simulink model "ADIA"  (R2018b)
settings: Solver=FixedStepDiscrete  StartTime=0.0  StopTime=10.0  FixedStep=0.02  RelTol=1e-3
undefined symbols (not defined in the file or in its folder): ACC_State_Active, ACC_State_BrakeOnly, ACC_State_Suspended, ACC_State_WaitingRise, ADAS_AEBBrakingProg, ADAS_DeclControlReq, ADAS_DriveOff, ADAS_ESCHoldReq_NotHold, ADASDecType_ACC, ADASDecType_AEB, ADIA_ACC_Acceleration_OOR_DecCount_C, ADIA_ACC_Acceleration_OOR_Duration_C, ADIA_ACC_Acceleration_OOR_IncCount_C, ADIA_ACC_Acceleration_OOR_LLim_C, ADIA_ACC_Acceleration_OOR_ULim_C, ADIA_ACC_AccelTrqReq_MixedDia_ULim_C, ADIA_ACC_AccelTrqReq_ULim_C, ADIA_ACC_Deceleration_Mixed_ULim_C, ADIA_ACC_Deceleration_OOR_DecCount_C, ADIA_ACC_Deceleration_OOR_Duration_C, ADIA_ACC_Deceleration_OOR_IncCount_C, ADIA_ACC_Deceleration_OOR_LLim_C, ADIA_ACC_Deceleration_OOR_ULim_C, ADIA_ACC_DriveOff_Distance_C, ADIA_ACC_DriveOff_TimeLim_C, ADIA_ACC_ReqMixed_DecCount_C, ADIA_ACC_ReqMixed_Duration_C, ADIA_ACC_ReqMixed_IncCount_C, ADIA_AccPedalRaw_MaxLim_C, ADIA_AccPedalRaw_MinLim_C, ADIA_ADAS_HoldDecReq_Set_C, ADIA_ADAS_HoldRConfirm_TimeLim_C, ADIA_ADAS_HoldVehSpd_Lim_C, ADIA_AEB_VehSpdDec_LLim_C, ADIA_AEB_VehSpdDec_ULim_C, ADIA_ASWFault_OvrdEn_C, ADIA_ASWFault_OvrdValue_C, ADIA_BatteryOutOfRange_DecCount_C, ADIA_BatteryOutOfRange_Duration_C, ADIA_BatteryOutOfRange_IncCount_C, ADIA_BattVolt_MaxLim_C, ADIA_BattVolt_MinLim_C, ADIA_BCM3_33C_InvBrkLight_DecCount_C, ADIA_BCM3_33C_InvBrkLight_Duration_C, ADIA_BCM3_33C_InvBrkLight_IncCount_C, ADIA_BCM_BattVolt_OvrdEn_C, ADIA_BCM_BattVolt_OvrdVal_C, ADIA_BCM_BrakeLampStaus_OvrdEn_C, ADIA_BCM_BrakeLampStaus_OvrdVal_C, ADIA_BCM_CHMSLStaus_OvrdEn_C, ADIA_BCM_CHMSLStaus_OvrdVal_C, ADIA_BCM_LeftTurnSwSt_OvrdEn_C, ADIA_BCM_LeftTurnSwSt_OvrdVal_C, ADIA_BCM_RightTurnSwSt_OvrdEn_C, ADIA_BCM_RightTurnSwSt_OvrdVal_C, ADIA_BCM_TurnSwFailure_DecCount_C, ADIA_BCM_TurnSwFailure_Duration_C, ADIA_BCM_TurnSwFailure_IncCount_C, ADIA_BSWFault_Ignore_C, ADIA_BSWFault_OvrdEn_C ... (+281)
libraries: simulink x208
(part 7 of 10)

== system ADIA/ADAS_Diagnostics/Diagnostics_Processing/Rationality_Diagnostics/ESC3_121_InvOorVehStand/Counter&Latch ==
  incrcondition : Inport
  incrvalue : Inport  Port=2
  decrcondition : Inport  Port=3
  decvalue : Inport  Port=4
  maxlimit : Inport  Port=5
  reset : Inport  Port=6
  LatchResetCounterVal : Inport  Port=7
  "Latch " : Subsystem
  Relational Operator16 : RelationalOperator  Operator=<=  OutDataTypeStr=boolean  RndMeth=Simplest
  Timer1 : Subsystem
  Out1 : Outport
  wires:
  Timer1/2(counter_status) -> "Latch "/1(Input)
  Timer1/1(counter out) -> Relational Operator16/1
  LatchResetCounterVal/1 -> Relational Operator16/2
  incrcondition/1 -> Timer1/1(incrcondition)
  incrvalue/1 -> Timer1/2(incrvalue)
  Relational Operator16/1 -> "Latch "/2(Latch Reset)
  "Latch "/1(Output) -> Out1/1
  maxlimit/1 -> Timer1/5(maxlimit)
  decrcondition/1 -> Timer1/3(decrcondition)
  reset/1 -> Timer1/6(reset)
  decvalue/1 -> Timer1/4(decvalue)

== system ADIA/ADAS_Diagnostics/Diagnostics_Processing/Rationality_Diagnostics/ESC5_122_InvOorLatAccel/Counter&Latch ==
  incrcondition : Inport
  incrvalue : Inport  Port=2
  decrcondition : Inport  Port=3
  decvalue : Inport  Port=4
  maxlimit : Inport  Port=5
  reset : Inport  Port=6
  LatchResetCounterVal : Inport  Port=7
  "Latch " : Subsystem
  Relational Operator16 : RelationalOperator  Operator=<=  OutDataTypeStr=boolean  RndMeth=Simplest
  Timer1 : Subsystem
  Out1 : Outport
  wires:
  Timer1/2(counter_status) -> "Latch "/1(Input)
  Timer1/1(counter out) -> Relational Operator16/1
  LatchResetCounterVal/1 -> Relational Operator16/2
  incrcondition/1 -> Timer1/1(incrcondition)
  incrvalue/1 -> Timer1/2(incrvalue)
  Relational Operator16/1 -> "Latch "/2(Latch Reset)
  "Latch "/1(Output) -> Out1/1
  maxlimit/1 -> Timer1/5(maxlimit)
  decrcondition/1 -> Timer1/3(decrcondition)
  reset/1 -> Timer1/6(reset)
  decvalue/1 -> Timer1/4(decvalue)

== system ADIA/ADAS_Diagnostics/Diagnostics_Processing/Rationality_Diagnostics/ESC5_122_InvOorLongiAccel/Counter&Latch ==
  incrcondition : Inport
  incrvalue : Inport  Port=2
  decrcondition : Inport  Port=3
  decvalue : Inport  Port=4
  maxlimit : Inport  Port=5
  reset : Inport  Port=6
  LatchResetCounterVal : Inport  Port=7
  "Latch " : Subsystem
  Relational Operator16 : RelationalOperator  Operator=<=  OutDataTypeStr=boolean  RndMeth=Simplest
  Timer1 : Subsystem
  Out1 : Outport
  wires:
  Timer1/2(counter_status) -> "Latch "/1(Input)
  Timer1/1(counter out) -> Relational Operator16/1
  LatchResetCounterVal/1 -> Relational Operator16/2
  incrcondition/1 -> Timer1/1(incrcondition)
  incrvalue/1 -> Timer1/2(incrvalue)
  Relational Operator16/1 -> "Latch "/2(Latch Reset)
  "Latch "/1(Output) -> Out1/1
  maxlimit/1 -> Timer1/5(maxlimit)
  decrcondition/1 -> Timer1/3(decrcondition)
  reset/1 -> Timer1/6(reset)
  decvalue/1 -> Timer1/4(decvalue)

== system ADIA/ADAS_Diagnostics/Diagnostics_Processing/Rationality_Diagnostics/ESC5_122_InvOorStaticSlope/Counter&Latch ==
  incrcondition : Inport
  incrvalue : Inport  Port=2
  decrcondition : Inport  Port=3
  decvalue : Inport  Port=4
  maxlimit : Inport  Port=5
  reset : Inport  Port=6
  LatchResetCounterVal : Inport  Port=7
  "Latch " : Subsystem
  Relational Operator16 : RelationalOperator  Operator=<=  OutDataTypeStr=boolean  RndMeth=Simplest
  Timer1 : Subsystem
  Out1 : Outport
  wires:
  Timer1/2(counter_status) -> "Latch "/1(Input)
  Timer1/1(counter out) -> Relational Operator16/1
  LatchResetCounterVal/1 -> Relational Operator16/2
  incrcondition/1 -> Timer1/1(incrcondition)
  incrvalue/1 -> Timer1/2(incrvalue)
  Relational Operator16/1 -> "Latch "/2(Latch Reset)
  "Latch "/1(Output) -> Out1/1
  maxlimit/1 -> Timer1/5(maxlimit)
  decrcondition/1 -> Timer1/3(decrcondition)
  reset/1 -> Timer1/6(reset)
  decvalue/1 -> Timer1/4(decvalue)

== system ADIA/ADAS_Diagnostics/Diagnostics_Processing/Rationality_Diagnostics/ESC5_122_InvOorYawRate/Counter&Latch ==
  incrcondition : Inport
  incrvalue : Inport  Port=2
  decrcondition : Inport  Port=3
  decvalue : Inport  Port=4
  maxlimit : Inport  Port=5
  reset : Inport  Port=6
  LatchResetCounterVal : Inport  Port=7
  "Latch " : Subsystem
  Relational Operator16 : RelationalOperator  Operator=<=  OutDataTypeStr=boolean  RndMeth=Simplest
  Timer1 : Subsystem
  Out1 : Outport
  wires:
  Timer1/2(counter_status) -> "Latch "/1(Input)
  Timer1/1(counter out) -> Relational Operator16/1
  LatchResetCounterVal/1 -> Relational Operator16/2
  incrcondition/1 -> Timer1/1(incrcondition)
  incrvalue/1 -> Timer1/2(incrvalue)
  Relational Operator16/1 -> "Latch "/2(Latch Reset)
  "Latch "/1(Output) -> Out1/1
  maxlimit/1 -> Timer1/5(maxlimit)
  decrcondition/1 -> Timer1/3(decrcondition)
  reset/1 -> Timer1/6(reset)
  decvalue/1 -> Timer1/4(decvalue)

== system ADIA/ADAS_Diagnostics/Diagnostics_Processing/Rationality_Diagnostics/ESC6_123_InvOorDynSlope/Counter&Latch ==
  incrcondition : Inport
  incrvalue : Inport  Port=2
  decrcondition : Inport  Port=3
  decvalue : Inport  Port=4
  maxlimit : Inport  Port=5
  reset : Inport  Port=6
  LatchResetCounterVal : Inport  Port=7
  "Latch " : Subsystem
  Relational Operator16 : RelationalOperator  Operator=<=  OutDataTypeStr=boolean  RndMeth=Simplest
  Timer1 : Subsystem
  Out1 : Outport
  wires:
  Timer1/2(counter_status) -> "Latch "/1(Input)
  Timer1/1(counter out) -> Relational Operator16/1
  LatchResetCounterVal/1 -> Relational Operator16/2
  incrcondition/1 -> Timer1/1(incrcondition)
  incrvalue/1 -> Timer1/2(incrvalue)
  Relational Operator16/1 -> "Latch "/2(Latch Reset)
  "Latch "/1(Output) -> Out1/1
  maxlimit/1 -> Timer1/5(maxlimit)
  decrcondition/1 -> Timer1/3(decrcondition)
  reset/1 -> Timer1/6(reset)
  decvalue/1 -> Timer1/4(decvalue)

== system ADIA/ADAS_Diagnostics/Diagnostics_Processing/Rationality_Diagnostics/ESC6_123_InvUnfilYawRate/Counter&Latch ==
  incrcondition : Inport
  incrvalue : Inport  Port=2
  decrcondition : Inport  Port=3
  decvalue : Inport  Port=4
  maxlimit : Inport  Port=5
  reset : Inport  Port=6
  LatchResetCounterVal : Inport  Port=7
  "Latch " : Subsystem
  Relational Operator16 : RelationalOperator  Operator=<=  OutDataTypeStr=boolean  RndMeth=Simplest
  Timer1 : Subsystem
  Out1 : Outport
  wires:
  Timer1/2(counter_status) -> "Latch "/1(Input)
  Timer1/1(counter out) -> Relational Operator16/1
  LatchResetCounterVal/1 -> Relational Operator16/2
  incrcondition/1 -> Timer1/1(incrcondition)
  incrvalue/1 -> Timer1/2(incrvalue)
  Relational Operator16/1 -> "Latch "/2(Latch Reset)
  "Latch "/1(Output) -> Out1/1
  maxlimit/1 -> Timer1/5(maxlimit)
  decrcondition/1 -> Timer1/3(decrcondition)
  reset/1 -> Timer1/6(reset)
  decvalue/1 -> Timer1/4(decvalue)

== system ADIA/ADAS_Diagnostics/Diagnostics_Processing/Rationality_Diagnostics/ESC6_123_InvVehDriDirec/Counter&Latch ==
  incrcondition : Inport
  incrvalue : Inport  Port=2
  decrcondition : Inport  Port=3
  decvalue : Inport  Port=4
  maxlimit : Inport  Port=5
  reset : Inport  Port=6
  LatchResetCounterVal : Inport  Port=7
  "Latch " : Subsystem
  Relational Operator16 : RelationalOperator  Operator=<=  OutDataTypeStr=boolean  RndMeth=Simplest
  Timer1 : Subsystem
  Out1 : Outport
  wires:
  Timer1/2(counter_status) -> "Latch "/1(Input)
  Timer1/1(counter out) -> Relational Operator16/1
  LatchResetCounterVal/1 -> Relational Operator16/2
  incrcondition/1 -> Timer1/1(incrcondition)
  incrvalue/1 -> Timer1/2(incrvalue)
  Relational Operator16/1 -> "Latch "/2(Latch Reset)
  "Latch "/1(Output) -> Out1/1
  maxlimit/1 -> Timer1/5(maxlimit)
  decrcondition/1 -> Timer1/3(decrcondition)
  reset/1 -> Timer1/6(reset)
  decvalue/1 -> Timer1/4(decvalue)

== system ADIA/ADAS_Diagnostics/Diagnostics_Processing/Rationality_Diagnostics/ESC6_123_InvVehHoldStas/Counter&Latch ==
  incrcondition : Inport
  incrvalue : Inport  Port=2
  decrcondition : Inport  Port=3
  decvalue : Inport  Port=4
  maxlimit : Inport  Port=5
  reset : Inport  Port=6
  LatchResetCounterVal : Inport  Port=7
  "Latch " : Subsystem
  Relational Operator16 : RelationalOperator  Operator=<=  OutDataTypeStr=boolean  RndMeth=Simplest
  Timer1 : Subsystem
  Out1 : Outport
  wires:
  Timer1/2(counter_status) -> "Latch "/1(Input)
  Timer1/1(counter out) -> Relational Operator16/1
  LatchResetCounterVal/1 -> Relational Operator16/2
  incrcondition/1 -> Timer1/1(incrcondition)
  incrvalue/1 -> Timer1/2(incrvalue)
  Relational Operator16/1 -> "Latch "/2(Latch Reset)
  "Latch "/1(Output) -> Out1/1
  maxlimit/1 -> Timer1/5(maxlimit)
  decrcondition/1 -> Timer1/3(decrcondition)
  reset/1 -> Timer1/6(reset)
  decvalue/1 -> Timer1/4(decvalue)

== system ADIA/ADAS_Diagnostics/Diagnostics_Processing/Rationality_Diagnostics/FRadar_FaultState/Counter&Latch ==
  incrcondition : Inport
  incrvalue : Inport  Port=2
  decrcondition : Inport  Port=3
  decvalue : Inport  Port=4
  maxlimit : Inport  Port=5
  reset : Inport  Port=6
  LatchResetCounterVal : Inport  Port=7
  "Latch " : Subsystem
  Relational Operator16 : RelationalOperator  Operator=<=  OutDataTypeStr=boolean  RndMeth=Simplest
  Timer1 : Subsystem
  Out1 : Outport
  wires:
  Timer1/2(counter_status) -> "Latch "/1(Input)
  Timer1/1(counter out) -> Relational Operator16/1
  LatchResetCounterVal/1 -> Relational Operator16/2
  incrcondition/1 -> Timer1/1(incrcondition)
  incrvalue/1 -> Timer1/2(incrvalue)
  Relational Operator16/1 -> "Latch "/2(Latch Reset)
  "Latch "/1(Output) -> Out1/1
  maxlimit/1 -> Timer1/5(maxlimit)
  decrcondition/1 -> Timer1/3(decrcondition)
  reset/1 -> Timer1/6(reset)
  decvalue/1 -> Timer1/4(decvalue)

== system ADIA/ADAS_Diagnostics/Diagnostics_Processing/Rationality_Diagnostics/MP5_366_OorAEBButton/Counter&Latch ==
  incrcondition : Inport
  incrvalue : Inport  Port=2
  decrcondition : Inport  Port=3
  decvalue : Inport  Port=4
  maxlimit : Inport  Port=5
  reset : Inport  Port=6
  LatchResetCounterVal : Inport  Port=7
  "Latch " : Subsystem
  Relational Operator16 : RelationalOperator  Operator=<=  OutDataTypeStr=boolean  RndMeth=Simplest
  Timer1 : Subsystem
  Out1 : Outport
  wires:
  Timer1/2(counter_status) -> "Latch "/1(Input)
  Timer1/1(counter out) -> Relational Operator16/1
  LatchResetCounterVal/1 -> Relational Operator16/2
  incrcondition/1 -> Timer1/1(incrcondition)
  incrvalue/1 -> Timer1/2(incrvalue)
  Relational Operator16/1 -> "Latch "/2(Latch Reset)
  "Latch "/1(Output) -> Out1/1
  maxlimit/1 -> Timer1/5(maxlimit)
  decrcondition/1 -> Timer1/3(decrcondition)
  reset/1 -> Timer1/6(reset)
  decvalue/1 -> Timer1/4(decvalue)

== system ADIA/ADAS_Diagnostics/Diagnostics_Processing/Rationality_Diagnostics/MP5_366_OorFCWButton/Counter&Latch ==
  incrcondition : Inport
  incrvalue : Inport  Port=2
  decrcondition : Inport  Port=3
  decvalue : Inport  Port=4
  maxlimit : Inport  Port=5
  reset : Inport  Port=6
  LatchResetCounterVal : Inport  Port=7
  "Latch " : Subsystem
  Relational Operator16 : RelationalOperator  Operator=<=  OutDataTypeStr=boolean  RndMeth=Simplest
  Timer1 : Subsystem
  Out1 : Outport
  wires:
  Timer1/2(counter_status) -> "Latch "/1(Input)
  Timer1/1(counter out) -> Relational Operator16/1
  LatchResetCounterVal/1 -> Relational Operator16/2
  incrcondition/1 -> Timer1/1(incrcondition)
  incrvalue/1 -> Timer1/2(incrvalue)
  Relational Operator16/1 -> "Latch "/2(Latch Reset)
  "Latch "/1(Output) -> Out1/1
  maxlimit/1 -> Timer1/5(maxlimit)
  decrcondition/1 -> Timer1/3(decrcondition)
  reset/1 -> Timer1/6(reset)
  decvalue/1 -> Timer1/4(decvalue)

== system ADIA/ADAS_Diagnostics/Diagnostics_Processing/Rationality_Diagnostics/MP5_413_OorISAMode/Counter&Latch ==
  incrcondition : Inport
  incrvalue : Inport  Port=2
  decrcondition : Inport  Port=3
  decvalue : Inport  Port=4
  maxlimit : Inport  Port=5
  reset : Inport  Port=6
  LatchResetCounterVal : Inport  Port=7
  "Latch " : Subsystem
  Relational Operator16 : RelationalOperator  Operator=<=  OutDataTypeStr=boolean  RndMeth=Simplest
  Timer1 : Subsystem
  Out1 : Outport
  wires:
  Timer1/2(counter_status) -> "Latch "/1(Input)
  Timer1/1(counter out) -> Relational Operator16/1
  LatchResetCounterVal/1 -> Relational Operator16/2
  incrcondition/1 -> Timer1/1(incrcondition)
  incrvalue/1 -> Timer1/2(incrvalue)
  Relational Operator16/1 -> "Latch "/2(Latch Reset)
  "Latch "/1(Output) -> Out1/1
  maxlimit/1 -> Timer1/5(maxlimit)
  decrcondition/1 -> Timer1/3(decrcondition)
  reset/1 -> Timer1/6(reset)
  decvalue/1 -> Timer1/4(decvalue)

== system ADIA/ADAS_Diagnostics/Diagnostics_Processing/Rationality_Diagnostics/MP5_413_OorLKAMode/Counter&Latch ==
  incrcondition : Inport
  incrvalue : Inport  Port=2
  decrcondition : Inport  Port=3
  decvalue : Inport  Port=4
  maxlimit : Inport  Port=5
  reset : Inport  Port=6
  LatchResetCounterVal : Inport  Port=7
  "Latch " : Subsystem
  Relational Operator16 : RelationalOperator  Operator=<=  OutDataTypeStr=boolean  RndMeth=Simplest
  Timer1 : Subsystem
  Out1 : Outport
  wires:
  Timer1/2(counter_status) -> "Latch "/1(Input)
  Timer1/1(counter out) -> Relational Operator16/1
  LatchResetCounterVal/1 -> Relational Operator16/2
  incrcondition/1 -> Timer1/1(incrcondition)
  incrvalue/1 -> Timer1/2(incrvalue)
  Relational Operator16/1 -> "Latch "/2(Latch Reset)
  "Latch "/1(Output) -> Out1/1
  maxlimit/1 -> Timer1/5(maxlimit)
  decrcondition/1 -> Timer1/3(decrcondition)
  reset/1 -> Timer1/6(reset)
  decvalue/1 -> Timer1/4(decvalue)

== system ADIA/ADAS_Diagnostics/Diagnostics_Processing/Rationality_Diagnostics/SAS_A5_InvOorSteAngle/Counter&Latch ==
  incrcondition : Inport
  incrvalue : Inport  Port=2
  decrcondition : Inport  Port=3
  decvalue : Inport  Port=4
  maxlimit : Inport  Port=5
  reset : Inport  Port=6
  LatchResetCounterVal : Inport  Port=7
  "Latch " : Subsystem
  Relational Operator16 : RelationalOperator  Operator=<=  OutDataTypeStr=boolean  RndMeth=Simplest
  Timer1 : Subsystem
  Out1 : Outport
  wires:
  Timer1/2(counter_status) -> "Latch "/1(Input)
  Timer1/1(counter out) -> Relational Operator16/1
  LatchResetCounterVal/1 -> Relational Operator16/2
  incrcondition/1 -> Timer1/1(incrcondition)
  incrvalue/1 -> Timer1/2(incrvalue)
  Relational Operator16/1 -> "Latch "/2(Latch Reset)
  "Latch "/1(Output) -> Out1/1
  maxlimit/1 -> Timer1/5(maxlimit)
  decrcondition/1 -> Timer1/3(decrcondition)
  reset/1 -> Timer1/6(reset)
  decvalue/1 -> Timer1/4(decvalue)

== system ADIA/ADAS_Diagnostics/Diagnostics_Processing/Rationality_Diagnostics/SAS_A5_InvRotSpeed/Counter&Latch ==
  incrcondition : Inport
  incrvalue : Inport  Port=2
  decrcondition : Inport  Port=3
  decvalue : Inport  Port=4
  maxlimit : Inport  Port=5
  reset : Inport  Port=6
  LatchResetCounterVal : Inport  Port=7
  "Latch " : Subsystem
  Relational Operator16 : RelationalOperator  Operator=<=  OutDataTypeStr=boolean  RndMeth=Simplest
  Timer1 : Subsystem
  Out1 : Outport
  wires:
  Timer1/2(counter_status) -> "Latch "/1(Input)
  Timer1/1(counter out) -> Relational Operator16/1
  LatchResetCounterVal/1 -> Relational Operator16/2
  incrcondition/1 -> Timer1/1(incrcondition)
  incrvalue/1 -> Timer1/2(incrvalue)
  Relational Operator16/1 -> "Latch "/2(Latch Reset)
  "Latch "/1(Output) -> Out1/1
  maxlimit/1 -> Timer1/5(maxlimit)
  decrcondition/1 -> Timer1/3(decrcondition)
  reset/1 -> Timer1/6(reset)
  decvalue/1 -> Timer1/4(decvalue)

== system ADIA/ADAS_Diagnostics/Diagnostics_Processing/Rationality_Diagnostics/SCC_309_OorACCButton/Counter&Latch ==
  incrcondition : Inport
  incrvalue : Inport  Port=2
  decrcondition : Inport  Port=3
  decvalue : Inport  Port=4
  maxlimit : Inport  Port=5
  reset : Inport  Port=6
  LatchResetCounterVal : Inport  Port=7
  "Latch " : Subsystem
  Relational Operator16 : RelationalOperator  Operator=<=  OutDataTypeStr=boolean  RndMeth=Simplest
  Timer1 : Subsystem
  Out1 : Outport
  wires:
  Timer1/2(counter_status) -> "Latch "/1(Input)
  Timer1/1(counter out) -> Relational Operator16/1
  LatchResetCounterVal/1 -> Relational Operator16/2
  incrcondition/1 -> Timer1/1(incrcondition)
  incrvalue/1 -> Timer1/2(incrvalue)
  Relational Operator16/1 -> "Latch "/2(Latch Reset)
  "Latch "/1(Output) -> Out1/1
  maxlimit/1 -> Timer1/5(maxlimit)
  decrcondition/1 -> Timer1/3(decrcondition)
  reset/1 -> Timer1/6(reset)
  decvalue/1 -> Timer1/4(decvalue)

== system ADIA/ADAS_Diagnostics/Diagnostics_Processing/Rationality_Diagnostics/Subsystem1/Counter&Latch ==
  incrcondition : Inport
  incrvalue : Inport  Port=2
  decrcondition : Inport  Port=3
  decvalue : Inport  Port=4
  maxlimit : Inport  Port=5
  reset : Inport  Port=6
  LatchResetCounterVal : Inport  Port=7
  "Latch " : Subsystem
  Relational Operator16 : RelationalOperator  Operator=<=  OutDataTypeStr=boolean  RndMeth=Simplest
  Timer1 : Subsystem
  Out1 : Outport
  wires:
  Timer1/2(counter_status) -> "Latch "/1(Input)
  Timer1/1(counter out) -> Relational Operator16/1
  LatchResetCounterVal/1 -> Relational Operator16/2
  incrcondition/1 -> Timer1/1(incrcondition)
  incrvalue/1 -> Timer1/2(incrvalue)
  Relational Operator16/1 -> "Latch "/2(Latch Reset)
  "Latch "/1(Output) -> Out1/1
  maxlimit/1 -> Timer1/5(maxlimit)
  decrcondition/1 -> Timer1/3(decrcondition)
  reset/1 -> Timer1/6(reset)
  decvalue/1 -> Timer1/4(decvalue)

== system ADIA/ADAS_Diagnostics/Diagnostics_Processing/Rationality_Diagnostics/Subsystem2/Counter&Latch ==
  incrcondition : Inport
  incrvalue : Inport  Port=2
  decrcondition : Inport  Port=3
  decvalue : Inport  Port=4
  maxlimit : Inport  Port=5
  reset : Inport  Port=6
  LatchResetCounterVal : Inport  Port=7
  "Latch " : Subsystem
  Relational Operator16 : RelationalOperator  Operator=<=  OutDataTypeStr=boolean  RndMeth=Simplest
  Timer1 : Subsystem
  Out1 : Outport
  wires:
  Timer1/2(counter_status) -> "Latch "/1(Input)
  Timer1/1(counter out) -> Relational Operator16/1
  LatchResetCounterVal/1 -> Relational Operator16/2
  incrcondition/1 -> Timer1/1(incrcondition)
  incrvalue/1 -> Timer1/2(incrvalue)
  Relational Operator16/1 -> "Latch "/2(Latch Reset)
  "Latch "/1(Output) -> Out1/1
  maxlimit/1 -> Timer1/5(maxlimit)
  decrcondition/1 -> Timer1/3(decrcondition)
  reset/1 -> Timer1/6(reset)
  decvalue/1 -> Timer1/4(decvalue)

== system ADIA/ADAS_Diagnostics/Diagnostics_Processing/Rationality_Diagnostics/Subsystem3/Counter&Latch ==
  incrcondition : Inport
  incrvalue : Inport  Port=2
  decrcondition : Inport  Port=3
  decvalue : Inport  Port=4
  maxlimit : Inport  Port=5
  reset : Inport  Port=6
  LatchResetCounterVal : Inport  Port=7
  "Latch " : Subsystem
  Relational Operator16 : RelationalOperator  Operator=<=  OutDataTypeStr=boolean  RndMeth=Simplest
  Timer1 : Subsystem
  Out1 : Outport
  wires:
  Timer1/2(counter_status) -> "Latch "/1(Input)
  Timer1/1(counter out) -> Relational Operator16/1
  LatchResetCounterVal/1 -> Relational Operator16/2
  incrcondition/1 -> Timer1/1(incrcondition)
  incrvalue/1 -> Timer1/2(incrvalue)
  Relational Operator16/1 -> "Latch "/2(Latch Reset)
  "Latch "/1(Output) -> Out1/1
  maxlimit/1 -> Timer1/5(maxlimit)
  decrcondition/1 -> Timer1/3(decrcondition)
  reset/1 -> Timer1/6(reset)
  decvalue/1 -> Timer1/4(decvalue)

== system ADIA/ADAS_Diagnostics/Diagnostics_Processing/Rationality_Diagnostics/TCU1_93_InvOorGear/Counter&Latch ==
  incrcondition : Inport
  incrvalue : Inport  Port=2
  decrcondition : Inport  Port=3
  decvalue : Inport  Port=4
  maxlimit : Inport  Port=5
  reset : Inport  Port=6
  LatchResetCounterVal : Inport  Port=7
  "Latch " : Subsystem
  Relational Operator16 : RelationalOperator  Operator=<=  OutDataTypeStr=boolean  RndMeth=Simplest
  Timer1 : Subsystem
  Out1 : Outport
  wires:
  Timer1/2(counter_status) -> "Latch "/1(Input)
  Timer1/1(counter out) -> Relational Operator16/1
  LatchResetCounterVal/1 -> Relational Operator16/2
  incrcondition/1 -> Timer1/1(incrcondition)
  incrvalue/1 -> Timer1/2(incrvalue)
  Relational Operator16/1 -> "Latch "/2(Latch Reset)
  "Latch "/1(Output) -> Out1/1
  maxlimit/1 -> Timer1/5(maxlimit)
  decrcondition/1 -> Timer1/3(decrcondition)
  reset/1 -> Timer1/6(reset)
  decvalue/1 -> Timer1/4(decvalue)

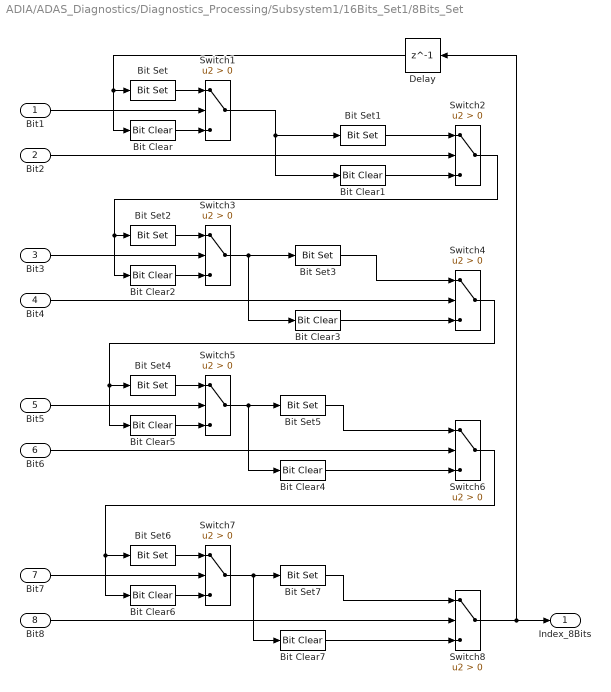
== system ADIA/ADAS_Diagnostics/Diagnostics_Processing/Subsystem1/16Bits_Set1/8Bits_Set ==
  Bit1 : Inport  OutDataTypeStr=boolean
  Bit2 : Inport  Port=2  OutDataTypeStr=boolean
  Bit3 : Inport  Port=3  OutDataTypeStr=boolean
  Bit4 : Inport  Port=4  OutDataTypeStr=boolean
  Bit5 : Inport  Port=5  OutDataTypeStr=boolean
  Bit6 : Inport  Port=6  OutDataTypeStr=boolean
  Bit7 : Inport  Port=7  OutDataTypeStr=boolean
  Bit8 : Inport  Port=8  OutDataTypeStr=boolean
  Bit Clear : simulink/Logic and Bit Operations/Bit Clear  iBit=0
      settings: SourceProductName=Simulink  SourceProductBaseCode=SL
  Bit Clear1 : simulink/Logic and Bit Operations/Bit Clear  iBit=1
      settings: SourceProductName=Simulink  SourceProductBaseCode=SL
  Bit Clear2 : simulink/Logic and Bit Operations/Bit Clear  iBit=2
      settings: SourceProductName=Simulink  SourceProductBaseCode=SL
  Bit Clear3 : simulink/Logic and Bit Operations/Bit Clear  iBit=3
      settings: SourceProductName=Simulink  SourceProductBaseCode=SL
  Bit Clear4 : simulink/Logic and Bit Operations/Bit Clear  iBit=5
      settings: SourceProductName=Simulink  SourceProductBaseCode=SL
  Bit Clear5 : simulink/Logic and Bit Operations/Bit Clear  iBit=4
      settings: SourceProductName=Simulink  SourceProductBaseCode=SL
  Bit Clear6 : simulink/Logic and Bit Operations/Bit Clear  iBit=6
      settings: SourceProductName=Simulink  SourceProductBaseCode=SL
  Bit Clear7 : simulink/Logic and Bit Operations/Bit Clear  iBit=7
      settings: SourceProductName=Simulink  SourceProductBaseCode=SL
  Bit Set : simulink/Logic and Bit Operations/Bit Set  iBit=0
      settings: SourceProductName=Simulink  SourceProductBaseCode=SL
  Bit Set1 : simulink/Logic and Bit Operations/Bit Set  iBit=1
      settings: SourceProductName=Simulink  SourceProductBaseCode=SL
  Bit Set2 : simulink/Logic and Bit Operations/Bit Set  iBit=2
      settings: SourceProductName=Simulink  SourceProductBaseCode=SL
  Bit Set3 : simulink/Logic and Bit Operations/Bit Set  iBit=3
      settings: SourceProductName=Simulink  SourceProductBaseCode=SL
  Bit Set4 : simulink/Logic and Bit Operations/Bit Set  iBit=4
      settings: SourceProductName=Simulink  SourceProductBaseCode=SL
  Bit Set5 : simulink/Logic and Bit Operations/Bit Set  iBit=5
      settings: SourceProductName=Simulink  SourceProductBaseCode=SL
  Bit Set6 : simulink/Logic and Bit Operations/Bit Set  iBit=6
      settings: SourceProductName=Simulink  SourceProductBaseCode=SL
  Bit Set7 : simulink/Logic and Bit Operations/Bit Set  iBit=7
      settings: SourceProductName=Simulink  SourceProductBaseCode=SL
  Delay : Delay  DelayLength=1  InitialCondition=0
  Switch{1..8} (8 alike) : Switch  Criteria=u2 > Threshold
  Index_8Bits : Outport  OutDataTypeStr=uint8
  wires:
  Bit Clear7/1 -> Switch8/3
  Bit Clear6/1 -> Switch7/3
  Bit Clear5/1 -> Switch5/3
  Bit Clear4/1 -> Switch6/3
  Bit Clear3/1 -> Switch4/3
  Bit Clear2/1 -> Switch3/3
  Bit Clear1/1 -> Switch2/3
  Bit Clear/1 -> Switch1/3
  Bit Set4/1 -> Switch5/1
  Bit Set2/1 -> Switch3/1
  Switch4/1 -> Bit Set4/1, Bit Clear5/1
  Switch6/1 -> Bit Set6/1, Bit Clear6/1
  Bit Set5/1 -> Switch6/1
  Switch7/1 -> Bit Set7/1, Bit Clear7/1
  Switch2/1 -> Bit Set2/1, Bit Clear2/1
  Bit Set3/1 -> Switch4/1
  Bit Set/1 -> Switch1/1
  Switch3/1 -> Bit Set3/1, Bit Clear3/1
  Bit7/1 -> Switch7/2
  Bit8/1 -> Switch8/2
  Bit Set6/1 -> Switch7/1
  Bit5/1 -> Switch5/2
  Bit6/1 -> Switch6/2
  Bit3/1 -> Switch3/2
  Bit Set1/1 -> Switch2/1
  Delay/1 -> Bit Set/1, Bit Clear/1
  Switch5/1 -> Bit Set5/1, Bit Clear4/1
  Bit2/1 -> Switch2/2
  Switch1/1 -> Bit Set1/1, Bit Clear1/1
  Switch8/1 -> Delay/1, Index_8Bits/1
  Bit4/1 -> Switch4/2
  Bit1/1 -> Switch1/2
  Bit Set7/1 -> Switch8/1

== system ADIA/ADAS_Diagnostics/Diagnostics_Processing/Subsystem1/16Bits_Set1/8Bits_Set1 ==
  Bit1 : Inport  OutDataTypeStr=boolean
  Bit2 : Inport  Port=2  OutDataTypeStr=boolean
  Bit3 : Inport  Port=3  OutDataTypeStr=boolean
  Bit4 : Inport  Port=4  OutDataTypeStr=boolean
  Bit5 : Inport  Port=5  OutDataTypeStr=boolean
  Bit6 : Inport  Port=6  OutDataTypeStr=boolean
  Bit7 : Inport  Port=7  OutDataTypeStr=boolean
  Bit8 : Inport  Port=8  OutDataTypeStr=boolean
  Bit Clear : simulink/Logic and Bit Operations/Bit Clear  iBit=0
      settings: SourceProductName=Simulink  SourceProductBaseCode=SL
  Bit Clear1 : simulink/Logic and Bit Operations/Bit Clear  iBit=1
      settings: SourceProductName=Simulink  SourceProductBaseCode=SL
  Bit Clear2 : simulink/Logic and Bit Operations/Bit Clear  iBit=2
      settings: SourceProductName=Simulink  SourceProductBaseCode=SL
  Bit Clear3 : simulink/Logic and Bit Operations/Bit Clear  iBit=3
      settings: SourceProductName=Simulink  SourceProductBaseCode=SL
  Bit Clear4 : simulink/Logic and Bit Operations/Bit Clear  iBit=5
      settings: SourceProductName=Simulink  SourceProductBaseCode=SL
  Bit Clear5 : simulink/Logic and Bit Operations/Bit Clear  iBit=4
      settings: SourceProductName=Simulink  SourceProductBaseCode=SL
  Bit Clear6 : simulink/Logic and Bit Operations/Bit Clear  iBit=6
      settings: SourceProductName=Simulink  SourceProductBaseCode=SL
  Bit Clear7 : simulink/Logic and Bit Operations/Bit Clear  iBit=7
      settings: SourceProductName=Simulink  SourceProductBaseCode=SL
  Bit Set : simulink/Logic and Bit Operations/Bit Set  iBit=0
      settings: SourceProductName=Simulink  SourceProductBaseCode=SL
  Bit Set1 : simulink/Logic and Bit Operations/Bit Set  iBit=1
      settings: SourceProductName=Simulink  SourceProductBaseCode=SL
  Bit Set2 : simulink/Logic and Bit Operations/Bit Set  iBit=2
      settings: SourceProductName=Simulink  SourceProductBaseCode=SL
  Bit Set3 : simulink/Logic and Bit Operations/Bit Set  iBit=3
      settings: SourceProductName=Simulink  SourceProductBaseCode=SL
  Bit Set4 : simulink/Logic and Bit Operations/Bit Set  iBit=4
      settings: SourceProductName=Simulink  SourceProductBaseCode=SL
  Bit Set5 : simulink/Logic and Bit Operations/Bit Set  iBit=5
      settings: SourceProductName=Simulink  SourceProductBaseCode=SL
  Bit Set6 : simulink/Logic and Bit Operations/Bit Set  iBit=6
      settings: SourceProductName=Simulink  SourceProductBaseCode=SL
  Bit Set7 : simulink/Logic and Bit Operations/Bit Set  iBit=7
      settings: SourceProductName=Simulink  SourceProductBaseCode=SL
  Delay : Delay  DelayLength=1  InitialCondition=0
  Switch{1..8} (8 alike) : Switch  Criteria=u2 > Threshold
  Index_8Bits : Outport  OutDataTypeStr=uint8
  wires:
  Bit Set7/1 -> Switch8/1
  Bit1/1 -> Switch1/2
  Bit4/1 -> Switch4/2
  Switch8/1 -> Index_8Bits/1, Delay/1
  Switch1/1 -> Bit Clear1/1, Bit Set1/1
  Bit2/1 -> Switch2/2
  Switch5/1 -> Bit Clear4/1, Bit Set5/1
  Delay/1 -> Bit Clear/1, Bit Set/1
  Bit Set1/1 -> Switch2/1
  Bit3/1 -> Switch3/2
  Bit6/1 -> Switch6/2
  Bit5/1 -> Switch5/2
  Bit Set6/1 -> Switch7/1
  Bit8/1 -> Switch8/2
  Bit7/1 -> Switch7/2
  Switch3/1 -> Bit Clear3/1, Bit Set3/1
  Bit Set/1 -> Switch1/1
  Bit Set3/1 -> Switch4/1
  Switch2/1 -> Bit Clear2/1, Bit Set2/1
  Switch7/1 -> Bit Clear7/1, Bit Set7/1
  Bit Set5/1 -> Switch6/1
  Switch6/1 -> Bit Clear6/1, Bit Set6/1
  Switch4/1 -> Bit Clear5/1, Bit Set4/1
  Bit Set2/1 -> Switch3/1
  Bit Set4/1 -> Switch5/1
  Bit Clear/1 -> Switch1/3
  Bit Clear1/1 -> Switch2/3
  Bit Clear2/1 -> Switch3/3
  Bit Clear3/1 -> Switch4/3
  Bit Clear4/1 -> Switch6/3
  Bit Clear5/1 -> Switch5/3
  Bit Clear6/1 -> Switch7/3
  Bit Clear7/1 -> Switch8/3

== system ADIA/ADAS_Diagnostics/Diagnostics_Processing/Subsystem1/16Bits_Set2/8Bits_Set ==
  Bit0 : Inport  OutDataTypeStr=boolean
  Bit1 : Inport  Port=2  OutDataTypeStr=boolean
  Bit2 : Inport  Port=3  OutDataTypeStr=boolean
  Bit3 : Inport  Port=4  OutDataTypeStr=boolean
  Bit4 : Inport  Port=5  OutDataTypeStr=boolean
  Bit5 : Inport  Port=6  OutDataTypeStr=boolean
  Bit6 : Inport  Port=7  OutDataTypeStr=boolean
  Bit7 : Inport  Port=8  OutDataTypeStr=boolean
  Bit Clear : simulink/Logic and Bit Operations/Bit Clear  iBit=0
      settings: SourceProductName=Simulink  SourceProductBaseCode=SL
  Bit Clear1 : simulink/Logic and Bit Operations/Bit Clear  iBit=1
      settings: SourceProductName=Simulink  SourceProductBaseCode=SL
  Bit Clear2 : simulink/Logic and Bit Operations/Bit Clear  iBit=2
      settings: SourceProductName=Simulink  SourceProductBaseCode=SL
  Bit Clear3 : simulink/Logic and Bit Operations/Bit Clear  iBit=3
      settings: SourceProductName=Simulink  SourceProductBaseCode=SL
  Bit Clear4 : simulink/Logic and Bit Operations/Bit Clear  iBit=5
      settings: SourceProductName=Simulink  SourceProductBaseCode=SL
  Bit Clear5 : simulink/Logic and Bit Operations/Bit Clear  iBit=4
      settings: SourceProductName=Simulink  SourceProductBaseCode=SL
  Bit Clear6 : simulink/Logic and Bit Operations/Bit Clear  iBit=6
      settings: SourceProductName=Simulink  SourceProductBaseCode=SL
  Bit Clear7 : simulink/Logic and Bit Operations/Bit Clear  iBit=7
      settings: SourceProductName=Simulink  SourceProductBaseCode=SL
  Bit Set : simulink/Logic and Bit Operations/Bit Set  iBit=0
      settings: SourceProductName=Simulink  SourceProductBaseCode=SL
  Bit Set1 : simulink/Logic and Bit Operations/Bit Set  iBit=1
      settings: SourceProductName=Simulink  SourceProductBaseCode=SL
  Bit Set2 : simulink/Logic and Bit Operations/Bit Set  iBit=2
      settings: SourceProductName=Simulink  SourceProductBaseCode=SL
  Bit Set3 : simulink/Logic and Bit Operations/Bit Set  iBit=3
      settings: SourceProductName=Simulink  SourceProductBaseCode=SL
  Bit Set4 : simulink/Logic and Bit Operations/Bit Set  iBit=4
      settings: SourceProductName=Simulink  SourceProductBaseCode=SL
  Bit Set5 : simulink/Logic and Bit Operations/Bit Set  iBit=5
      settings: SourceProductName=Simulink  SourceProductBaseCode=SL
  Bit Set6 : simulink/Logic and Bit Operations/Bit Set  iBit=6
      settings: SourceProductName=Simulink  SourceProductBaseCode=SL
  Bit Set7 : simulink/Logic and Bit Operations/Bit Set  iBit=7
      settings: SourceProductName=Simulink  SourceProductBaseCode=SL
  Delay : Delay  DelayLength=1  InitialCondition=0
  Switch{1..8} (8 alike) : Switch  Criteria=u2 > Threshold
  Index_8Bits : Outport  OutDataTypeStr=uint8
  wires:
  Bit Set7/1 -> Switch8/1
  Bit0/1 -> Switch1/2
  Bit3/1 -> Switch4/2
  Switch8/1 -> Index_8Bits/1, Delay/1
  Switch1/1 -> Bit Clear1/1, Bit Set1/1
  Bit1/1 -> Switch2/2
  Switch5/1 -> Bit Clear4/1, Bit Set5/1
  Delay/1 -> Bit Clear/1, Bit Set/1
  Bit Set1/1 -> Switch2/1
  Bit2/1 -> Switch3/2
  Bit5/1 -> Switch6/2
  Bit4/1 -> Switch5/2
  Bit Set6/1 -> Switch7/1
  Bit7/1 -> Switch8/2
  Bit6/1 -> Switch7/2
  Switch3/1 -> Bit Clear3/1, Bit Set3/1
  Bit Set/1 -> Switch1/1
  Bit Set3/1 -> Switch4/1
  Switch2/1 -> Bit Clear2/1, Bit Set2/1
  Switch7/1 -> Bit Clear7/1, Bit Set7/1
  Bit Set5/1 -> Switch6/1
  Switch6/1 -> Bit Clear6/1, Bit Set6/1
  Switch4/1 -> Bit Clear5/1, Bit Set4/1
  Bit Set2/1 -> Switch3/1
  Bit Set4/1 -> Switch5/1
  Bit Clear/1 -> Switch1/3
  Bit Clear1/1 -> Switch2/3
  Bit Clear2/1 -> Switch3/3
  Bit Clear3/1 -> Switch4/3
  Bit Clear4/1 -> Switch6/3
  Bit Clear5/1 -> Switch5/3
  Bit Clear6/1 -> Switch7/3
  Bit Clear7/1 -> Switch8/3

== system ADIA/ADAS_Diagnostics/Diagnostics_Processing/Subsystem1/16Bits_Set2/8Bits_Set1 ==
  Bit0 : Inport  OutDataTypeStr=boolean
  Bit1 : Inport  Port=2  OutDataTypeStr=boolean
  Bit2 : Inport  Port=3  OutDataTypeStr=boolean
  Bit3 : Inport  Port=4  OutDataTypeStr=boolean
  Bit4 : Inport  Port=5  OutDataTypeStr=boolean
  Bit5 : Inport  Port=6  OutDataTypeStr=boolean
  Bit6 : Inport  Port=7  OutDataTypeStr=boolean
  Bit7 : Inport  Port=8  OutDataTypeStr=boolean
  Bit Clear : simulink/Logic and Bit Operations/Bit Clear  iBit=0
      settings: SourceProductName=Simulink  SourceProductBaseCode=SL
  Bit Clear1 : simulink/Logic and Bit Operations/Bit Clear  iBit=1
      settings: SourceProductName=Simulink  SourceProductBaseCode=SL
  Bit Clear2 : simulink/Logic and Bit Operations/Bit Clear  iBit=2
      settings: SourceProductName=Simulink  SourceProductBaseCode=SL
  Bit Clear3 : simulink/Logic and Bit Operations/Bit Clear  iBit=3
      settings: SourceProductName=Simulink  SourceProductBaseCode=SL
  Bit Clear4 : simulink/Logic and Bit Operations/Bit Clear  iBit=5
      settings: SourceProductName=Simulink  SourceProductBaseCode=SL
  Bit Clear5 : simulink/Logic and Bit Operations/Bit Clear  iBit=4
      settings: SourceProductName=Simulink  SourceProductBaseCode=SL
  Bit Clear6 : simulink/Logic and Bit Operations/Bit Clear  iBit=6
      settings: SourceProductName=Simulink  SourceProductBaseCode=SL
  Bit Clear7 : simulink/Logic and Bit Operations/Bit Clear  iBit=7
      settings: SourceProductName=Simulink  SourceProductBaseCode=SL
  Bit Set : simulink/Logic and Bit Operations/Bit Set  iBit=0
      settings: SourceProductName=Simulink  SourceProductBaseCode=SL
  Bit Set1 : simulink/Logic and Bit Operations/Bit Set  iBit=1
      settings: SourceProductName=Simulink  SourceProductBaseCode=SL
  Bit Set2 : simulink/Logic and Bit Operations/Bit Set  iBit=2
      settings: SourceProductName=Simulink  SourceProductBaseCode=SL
  Bit Set3 : simulink/Logic and Bit Operations/Bit Set  iBit=3
      settings: SourceProductName=Simulink  SourceProductBaseCode=SL
  Bit Set4 : simulink/Logic and Bit Operations/Bit Set  iBit=4
      settings: SourceProductName=Simulink  SourceProductBaseCode=SL
  Bit Set5 : simulink/Logic and Bit Operations/Bit Set  iBit=5
      settings: SourceProductName=Simulink  SourceProductBaseCode=SL
  Bit Set6 : simulink/Logic and Bit Operations/Bit Set  iBit=6
      settings: SourceProductName=Simulink  SourceProductBaseCode=SL
  Bit Set7 : simulink/Logic and Bit Operations/Bit Set  iBit=7
      settings: SourceProductName=Simulink  SourceProductBaseCode=SL
  Delay : Delay  DelayLength=1  InitialCondition=0
  Switch{1..8} (8 alike) : Switch  Criteria=u2 > Threshold
  Index_8Bits : Outport  OutDataTypeStr=uint8
  wires:
  Bit Clear7/1 -> Switch8/3
  Bit Clear6/1 -> Switch7/3
  Bit Clear5/1 -> Switch5/3
  Bit Clear4/1 -> Switch6/3
  Bit Clear3/1 -> Switch4/3
  Bit Clear2/1 -> Switch3/3
  Bit Clear1/1 -> Switch2/3
  Bit Clear/1 -> Switch1/3
  Bit Set4/1 -> Switch5/1
  Bit Set2/1 -> Switch3/1
  Switch4/1 -> Bit Set4/1, Bit Clear5/1
  Switch6/1 -> Bit Set6/1, Bit Clear6/1
  Bit Set5/1 -> Switch6/1
  Switch7/1 -> Bit Set7/1, Bit Clear7/1
  Switch2/1 -> Bit Set2/1, Bit Clear2/1
  Bit Set3/1 -> Switch4/1
  Bit Set/1 -> Switch1/1
  Switch3/1 -> Bit Set3/1, Bit Clear3/1
  Bit6/1 -> Switch7/2
  Bit7/1 -> Switch8/2
  Bit Set6/1 -> Switch7/1
  Bit4/1 -> Switch5/2
  Bit5/1 -> Switch6/2
  Bit2/1 -> Switch3/2
  Bit Set1/1 -> Switch2/1
  Delay/1 -> Bit Set/1, Bit Clear/1
  Switch5/1 -> Bit Set5/1, Bit Clear4/1
  Bit1/1 -> Switch2/2
  Switch1/1 -> Bit Set1/1, Bit Clear1/1
  Switch8/1 -> Delay/1, Index_8Bits/1
  Bit3/1 -> Switch4/2
  Bit0/1 -> Switch1/2
  Bit Set7/1 -> Switch8/1

== system ADIA/ADAS_Diagnostics/Diagnostics_Processing/Subsystem3/16Bits_Set/8Bits_Set ==
  Bit0 : Inport  OutDataTypeStr=boolean
  Bit1 : Inport  Port=2  OutDataTypeStr=boolean
  Bit2 : Inport  Port=3  OutDataTypeStr=boolean
  Bit3 : Inport  Port=4  OutDataTypeStr=boolean
  Bit4 : Inport  Port=5  OutDataTypeStr=boolean
  Bit5 : Inport  Port=6  OutDataTypeStr=boolean
  Bit6 : Inport  Port=7  OutDataTypeStr=boolean
  Bit7 : Inport  Port=8  OutDataTypeStr=boolean
  Bit Clear : simulink/Logic and Bit Operations/Bit Clear  iBit=0
      settings: SourceProductName=Simulink  SourceProductBaseCode=SL
  Bit Clear1 : simulink/Logic and Bit Operations/Bit Clear  iBit=1
      settings: SourceProductName=Simulink  SourceProductBaseCode=SL
  Bit Clear2 : simulink/Logic and Bit Operations/Bit Clear  iBit=2
      settings: SourceProductName=Simulink  SourceProductBaseCode=SL
  Bit Clear3 : simulink/Logic and Bit Operations/Bit Clear  iBit=3
      settings: SourceProductName=Simulink  SourceProductBaseCode=SL
  Bit Clear4 : simulink/Logic and Bit Operations/Bit Clear  iBit=5
      settings: SourceProductName=Simulink  SourceProductBaseCode=SL
  Bit Clear5 : simulink/Logic and Bit Operations/Bit Clear  iBit=4
      settings: SourceProductName=Simulink  SourceProductBaseCode=SL
  Bit Clear6 : simulink/Logic and Bit Operations/Bit Clear  iBit=6
      settings: SourceProductName=Simulink  SourceProductBaseCode=SL
  Bit Clear7 : simulink/Logic and Bit Operations/Bit Clear  iBit=7
      settings: SourceProductName=Simulink  SourceProductBaseCode=SL
  Bit Set : simulink/Logic and Bit Operations/Bit Set  iBit=0
      settings: SourceProductName=Simulink  SourceProductBaseCode=SL
  Bit Set1 : simulink/Logic and Bit Operations/Bit Set  iBit=1
      settings: SourceProductName=Simulink  SourceProductBaseCode=SL
  Bit Set2 : simulink/Logic and Bit Operations/Bit Set  iBit=2
      settings: SourceProductName=Simulink  SourceProductBaseCode=SL
  Bit Set3 : simulink/Logic and Bit Operations/Bit Set  iBit=3
      settings: SourceProductName=Simulink  SourceProductBaseCode=SL
  Bit Set4 : simulink/Logic and Bit Operations/Bit Set  iBit=4
      settings: SourceProductName=Simulink  SourceProductBaseCode=SL
  Bit Set5 : simulink/Logic and Bit Operations/Bit Set  iBit=5
      settings: SourceProductName=Simulink  SourceProductBaseCode=SL
  Bit Set6 : simulink/Logic and Bit Operations/Bit Set  iBit=6
      settings: SourceProductName=Simulink  SourceProductBaseCode=SL
  Bit Set7 : simulink/Logic and Bit Operations/Bit Set  iBit=7
      settings: SourceProductName=Simulink  SourceProductBaseCode=SL
  Delay : Delay  DelayLength=1  InitialCondition=0
  Switch{1..8} (8 alike) : Switch  Criteria=u2 > Threshold
  Index_8Bits : Outport  OutDataTypeStr=uint8
  wires:
  Bit Clear7/1 -> Switch8/3
  Bit Clear6/1 -> Switch7/3
  Bit Clear5/1 -> Switch5/3
  Bit Clear4/1 -> Switch6/3
  Bit Clear3/1 -> Switch4/3
  Bit Clear2/1 -> Switch3/3
  Bit Clear1/1 -> Switch2/3
  Bit Clear/1 -> Switch1/3
  Bit Set4/1 -> Switch5/1
  Bit Set2/1 -> Switch3/1
  Switch4/1 -> Bit Set4/1, Bit Clear5/1
  Switch6/1 -> Bit Set6/1, Bit Clear6/1
  Bit Set5/1 -> Switch6/1
  Switch7/1 -> Bit Set7/1, Bit Clear7/1
  Switch2/1 -> Bit Set2/1, Bit Clear2/1
  Bit Set3/1 -> Switch4/1
  Bit Set/1 -> Switch1/1
  Switch3/1 -> Bit Set3/1, Bit Clear3/1
  Bit6/1 -> Switch7/2
  Bit7/1 -> Switch8/2
  Bit Set6/1 -> Switch7/1
  Bit4/1 -> Switch5/2
  Bit5/1 -> Switch6/2
  Bit2/1 -> Switch3/2
  Bit Set1/1 -> Switch2/1
  Delay/1 -> Bit Set/1, Bit Clear/1
  Switch5/1 -> Bit Set5/1, Bit Clear4/1
  Bit1/1 -> Switch2/2
  Switch1/1 -> Bit Set1/1, Bit Clear1/1
  Switch8/1 -> Delay/1, Index_8Bits/1
  Bit3/1 -> Switch4/2
  Bit0/1 -> Switch1/2
  Bit Set7/1 -> Switch8/1

== system ADIA/ADAS_Diagnostics/Diagnostics_Processing/Subsystem3/16Bits_Set/8Bits_Set1 ==
  Bit0 : Inport  OutDataTypeStr=boolean
  Bit1 : Inport  Port=2  OutDataTypeStr=boolean
  Bit2 : Inport  Port=3  OutDataTypeStr=boolean
  Bit3 : Inport  Port=4  OutDataTypeStr=boolean
  Bit4 : Inport  Port=5  OutDataTypeStr=boolean
  Bit5 : Inport  Port=6  OutDataTypeStr=boolean
  Bit6 : Inport  Port=7  OutDataTypeStr=boolean
  Bit7 : Inport  Port=8  OutDataTypeStr=boolean
  Bit Clear : simulink/Logic and Bit Operations/Bit Clear  iBit=0
      settings: SourceProductName=Simulink  SourceProductBaseCode=SL
  Bit Clear1 : simulink/Logic and Bit Operations/Bit Clear  iBit=1
      settings: SourceProductName=Simulink  SourceProductBaseCode=SL
  Bit Clear2 : simulink/Logic and Bit Operations/Bit Clear  iBit=2
      settings: SourceProductName=Simulink  SourceProductBaseCode=SL
  Bit Clear3 : simulink/Logic and Bit Operations/Bit Clear  iBit=3
      settings: SourceProductName=Simulink  SourceProductBaseCode=SL
  Bit Clear4 : simulink/Logic and Bit Operations/Bit Clear  iBit=5
      settings: SourceProductName=Simulink  SourceProductBaseCode=SL
  Bit Clear5 : simulink/Logic and Bit Operations/Bit Clear  iBit=4
      settings: SourceProductName=Simulink  SourceProductBaseCode=SL
  Bit Clear6 : simulink/Logic and Bit Operations/Bit Clear  iBit=6
      settings: SourceProductName=Simulink  SourceProductBaseCode=SL
  Bit Clear7 : simulink/Logic and Bit Operations/Bit Clear  iBit=7
      settings: SourceProductName=Simulink  SourceProductBaseCode=SL
  Bit Set : simulink/Logic and Bit Operations/Bit Set  iBit=0
      settings: SourceProductName=Simulink  SourceProductBaseCode=SL
  Bit Set1 : simulink/Logic and Bit Operations/Bit Set  iBit=1
      settings: SourceProductName=Simulink  SourceProductBaseCode=SL
  Bit Set2 : simulink/Logic and Bit Operations/Bit Set  iBit=2
      settings: SourceProductName=Simulink  SourceProductBaseCode=SL
  Bit Set3 : simulink/Logic and Bit Operations/Bit Set  iBit=3
      settings: SourceProductName=Simulink  SourceProductBaseCode=SL
  Bit Set4 : simulink/Logic and Bit Operations/Bit Set  iBit=4
      settings: SourceProductName=Simulink  SourceProductBaseCode=SL
  Bit Set5 : simulink/Logic and Bit Operations/Bit Set  iBit=5
      settings: SourceProductName=Simulink  SourceProductBaseCode=SL
  Bit Set6 : simulink/Logic and Bit Operations/Bit Set  iBit=6
      settings: SourceProductName=Simulink  SourceProductBaseCode=SL
  Bit Set7 : simulink/Logic and Bit Operations/Bit Set  iBit=7
      settings: SourceProductName=Simulink  SourceProductBaseCode=SL
  Delay : Delay  DelayLength=1  InitialCondition=0
  Switch{1..8} (8 alike) : Switch  Criteria=u2 > Threshold
  Index_8Bits : Outport  OutDataTypeStr=uint8
  wires:
  Bit Set7/1 -> Switch8/1
  Bit0/1 -> Switch1/2
  Bit3/1 -> Switch4/2
  Switch8/1 -> Index_8Bits/1, Delay/1
  Switch1/1 -> Bit Clear1/1, Bit Set1/1
  Bit1/1 -> Switch2/2
  Switch5/1 -> Bit Clear4/1, Bit Set5/1
  Delay/1 -> Bit Clear/1, Bit Set/1
  Bit Set1/1 -> Switch2/1
  Bit2/1 -> Switch3/2
  Bit5/1 -> Switch6/2
  Bit4/1 -> Switch5/2
  Bit Set6/1 -> Switch7/1
  Bit7/1 -> Switch8/2
  Bit6/1 -> Switch7/2
  Switch3/1 -> Bit Clear3/1, Bit Set3/1
  Bit Set/1 -> Switch1/1
  Bit Set3/1 -> Switch4/1
  Switch2/1 -> Bit Clear2/1, Bit Set2/1
  Switch7/1 -> Bit Clear7/1, Bit Set7/1
  Bit Set5/1 -> Switch6/1
  Switch6/1 -> Bit Clear6/1, Bit Set6/1
  Switch4/1 -> Bit Clear5/1, Bit Set4/1
  Bit Set2/1 -> Switch3/1
  Bit Set4/1 -> Switch5/1
  Bit Clear/1 -> Switch1/3
  Bit Clear1/1 -> Switch2/3
  Bit Clear2/1 -> Switch3/3
  Bit Clear3/1 -> Switch4/3
  Bit Clear4/1 -> Switch6/3
  Bit Clear5/1 -> Switch5/3
  Bit Clear6/1 -> Switch7/3
  Bit Clear7/1 -> Switch8/3

== system ADIA/ADAS_Diagnostics/Diagnostics_Processing/Subsystem3/16Bits_Set1/8Bits_Set ==
  Bit1 : Inport  OutDataTypeStr=boolean
  Bit2 : Inport  Port=2  OutDataTypeStr=boolean
  Bit3 : Inport  Port=3  OutDataTypeStr=boolean
  Bit4 : Inport  Port=4  OutDataTypeStr=boolean
  Bit5 : Inport  Port=5  OutDataTypeStr=boolean
  Bit6 : Inport  Port=6  OutDataTypeStr=boolean
  Bit7 : Inport  Port=7  OutDataTypeStr=boolean
  Bit8 : Inport  Port=8  OutDataTypeStr=boolean
  Bit Clear : simulink/Logic and Bit Operations/Bit Clear  iBit=0
      settings: SourceProductName=Simulink  SourceProductBaseCode=SL
  Bit Clear1 : simulink/Logic and Bit Operations/Bit Clear  iBit=1
      settings: SourceProductName=Simulink  SourceProductBaseCode=SL
  Bit Clear2 : simulink/Logic and Bit Operations/Bit Clear  iBit=2
      settings: SourceProductName=Simulink  SourceProductBaseCode=SL
  Bit Clear3 : simulink/Logic and Bit Operations/Bit Clear  iBit=3
      settings: SourceProductName=Simulink  SourceProductBaseCode=SL
  Bit Clear4 : simulink/Logic and Bit Operations/Bit Clear  iBit=5
      settings: SourceProductName=Simulink  SourceProductBaseCode=SL
  Bit Clear5 : simulink/Logic and Bit Operations/Bit Clear  iBit=4
      settings: SourceProductName=Simulink  SourceProductBaseCode=SL
  Bit Clear6 : simulink/Logic and Bit Operations/Bit Clear  iBit=6
      settings: SourceProductName=Simulink  SourceProductBaseCode=SL
  Bit Clear7 : simulink/Logic and Bit Operations/Bit Clear  iBit=7
      settings: SourceProductName=Simulink  SourceProductBaseCode=SL
  Bit Set : simulink/Logic and Bit Operations/Bit Set  iBit=0
      settings: SourceProductName=Simulink  SourceProductBaseCode=SL
  Bit Set1 : simulink/Logic and Bit Operations/Bit Set  iBit=1
      settings: SourceProductName=Simulink  SourceProductBaseCode=SL
  Bit Set2 : simulink/Logic and Bit Operations/Bit Set  iBit=2
      settings: SourceProductName=Simulink  SourceProductBaseCode=SL
  Bit Set3 : simulink/Logic and Bit Operations/Bit Set  iBit=3
      settings: SourceProductName=Simulink  SourceProductBaseCode=SL
  Bit Set4 : simulink/Logic and Bit Operations/Bit Set  iBit=4
      settings: SourceProductName=Simulink  SourceProductBaseCode=SL
  Bit Set5 : simulink/Logic and Bit Operations/Bit Set  iBit=5
      settings: SourceProductName=Simulink  SourceProductBaseCode=SL
  Bit Set6 : simulink/Logic and Bit Operations/Bit Set  iBit=6
      settings: SourceProductName=Simulink  SourceProductBaseCode=SL
  Bit Set7 : simulink/Logic and Bit Operations/Bit Set  iBit=7
      settings: SourceProductName=Simulink  SourceProductBaseCode=SL
  Delay : Delay  DelayLength=1  InitialCondition=0
  Switch{1..8} (8 alike) : Switch  Criteria=u2 > Threshold
  Index_8Bits : Outport  OutDataTypeStr=uint8
  wires:
  Bit Set7/1 -> Switch8/1
  Bit1/1 -> Switch1/2
  Bit4/1 -> Switch4/2
  Switch8/1 -> Index_8Bits/1, Delay/1
  Switch1/1 -> Bit Clear1/1, Bit Set1/1
  Bit2/1 -> Switch2/2
  Switch5/1 -> Bit Clear4/1, Bit Set5/1
  Delay/1 -> Bit Clear/1, Bit Set/1
  Bit Set1/1 -> Switch2/1
  Bit3/1 -> Switch3/2
  Bit6/1 -> Switch6/2
  Bit5/1 -> Switch5/2
  Bit Set6/1 -> Switch7/1
  Bit8/1 -> Switch8/2
  Bit7/1 -> Switch7/2
  Switch3/1 -> Bit Clear3/1, Bit Set3/1
  Bit Set/1 -> Switch1/1
  Bit Set3/1 -> Switch4/1
  Switch2/1 -> Bit Clear2/1, Bit Set2/1
  Switch7/1 -> Bit Clear7/1, Bit Set7/1
  Bit Set5/1 -> Switch6/1
  Switch6/1 -> Bit Clear6/1, Bit Set6/1
  Switch4/1 -> Bit Clear5/1, Bit Set4/1
  Bit Set2/1 -> Switch3/1
  Bit Set4/1 -> Switch5/1
  Bit Clear/1 -> Switch1/3
  Bit Clear1/1 -> Switch2/3
  Bit Clear2/1 -> Switch3/3
  Bit Clear3/1 -> Switch4/3
  Bit Clear4/1 -> Switch6/3
  Bit Clear5/1 -> Switch5/3
  Bit Clear6/1 -> Switch7/3
  Bit Clear7/1 -> Switch8/3
